simulink model "seperator"  (R2021b)
settings: Solver=VariableStepAuto  StartTime=0.0  StopTime=100  RelTol=1e-3
settings Model: Creator=Edwar  LastModifiedBy=Edwar

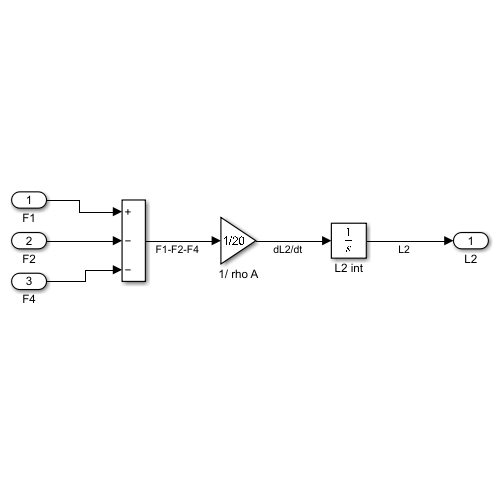
[thumbnail: Simulink's stored preview of the top-level diagram]
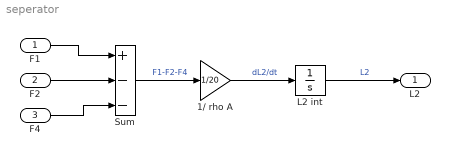
== system seperator ==
  F1 : Inport
  F2 : Inport  Port=2
  F4 : Inport  Port=3
  1/ rho A : Gain  Gain=1/20
  L2 int : Integrator
  Sum : Sum  Inputs=+--
  L2 : Outport
  wires:
  Sum/1 -> 1/ rho A/1  "F1-F2-F4"
  1/ rho A/1 -> L2 int/1  "dL2/dt"
  L2 int/1 -> L2/1  "L2"
  F4/1 -> Sum/3
  F2/1 -> Sum/2
  F1/1 -> Sum/1
